simulink subsystem "ControlerBA"  (R2023b)
settings: Solver=VariableStepAuto  StartTime=0.0  StopTime=10.0  RelTol=1e-3
settings Model: Creator=alumnos  LastModifiedBy=Usuario_UMA

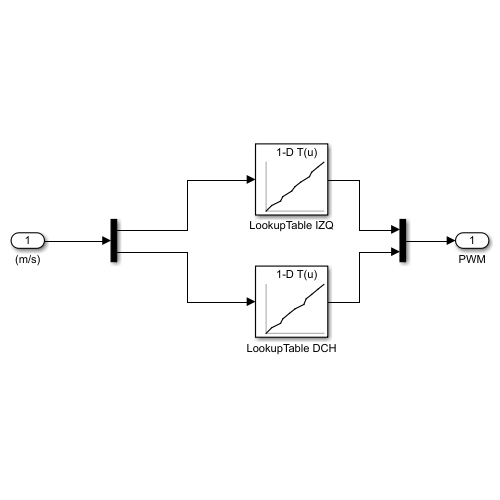
[thumbnail: Simulink's stored preview of the top-level diagram]
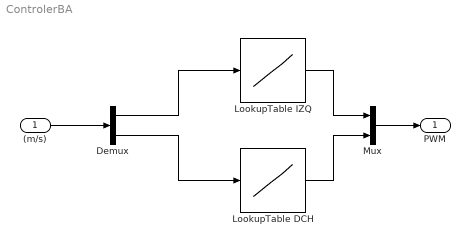
== system ControlerBA ==
  (m/s) : Inport
  Demux : Demux  Outputs=2
  LookupTable DCH : Lookup_n-D  NumberOfTableDimensions=1  BreakpointsForDimension1=[-0.82904052734375 -0.663215637207031 -0.414520263671875 -0.331619262695313 -0.165802001953125 0 0.248703002929688 0.33160400390625 0.497406005859375 0.663215637207031 0.829032897949219]  Table=[-255 -200.174957275391 -150.449981689453 -100.724998474121 -49.724983215332 0 49.724983215332 100.724998474121 150.450012207031 200.175018310547 255]  InternalRulePriority=Speed  RndMeth=Simplest
  LookupTable IZQ : Lookup_n-D  NumberOfTableDimensions=1  BreakpointsForDimension1=[-0.829032897949219 -0.663223266601563 -0.414505004882813 -0.331619262695313 -0.0829010009765625 0 0.165802001953125 0.414505004882813 0.497421264648438 0.663223266601563 0.829032897949219]  Table=[-255 -200.174957275391 -150.449981689453 -100.724998474121 -49.724983215332 0 49.724983215332 100.724998474121 150.450012207031 200.175018310547 255]  InternalRulePriority=Speed  RndMeth=Simplest
  Mux : Mux  Inputs=2
  PWM : Outport
  wires:
  (m/s)/1 -> Demux/1
  Demux/1 -> LookupTable IZQ/1
  Demux/2 -> LookupTable DCH/1
  LookupTable IZQ/1 -> Mux/1
  LookupTable DCH/1 -> Mux/2
  Mux/1 -> PWM/1
